simulink model "testSFunctionBuilder"  (R2016a)
settings: Solver=ode1  StartTime=0.0  StopTime=10  FixedStep=0.001  RelTol=1e-3
PostLoadFcn:
  | , if any(exist('dsrtsu_mdlpostloadfcn', 'file') == [2, 3, 6]), try dsrtsu_mdlpostloadfcn('Execute', bdroot); catch fprintf('Error in PostLoadFcn (dsrtsu_mdlpostloadfcn) for model "%s":\n %s\n', bdroot, lasterr); end, end,
settings Model: DSRTSU_INTERNAL_RTI_VER=490  DSRTSU_INTERNAL_RTI_TYPE=rti1401  RTICANMMDATA=struct('GeneralSetupData',struct('modelroot','Z:\Workspace\library\TestSFunctionBuilder','generalsettings',struct('filesettings',struct('destfolder',struct('Name','RTICANMM_FILES','Check',1),'buildfolder',struct('Name','.','Check',1),'AbsDestfolder',struct('Name','Z:\Workspace\library\TestSFunctionBuilder\RTICANMM_FILES'),'AbsBuildfolder',struct('Name','Z:\Workspace\library\TestSFunctionBuilder'))),'options',struct('addpaths',1,'rmpaths',1,'addtrcexclusion',logical(1),'cannavigator',struct('checkmonitoring',0),'show_usrtrc',0,'use_usrtrc',0),'advanced',struct('options',[1 1 1 1 1 1 1 1 1 1 1 1 1 1 1 1 1 1 1 1 1 1 1 1 1 1 1 1 1 1 1 1 1 1 1 1 1 1 1 1 1 1 1 1 1 1 1 1 1 1 1 1 1 1 1 1 1 1 1 1 1 1 1 1 1 1 1 1 1 1 1 1 1 1 1 1 1 1 1 1 1 1 1 1 1 1 1 1 1 1 1 1 1 1 1 1 1 1 1 1]),'MPSetup',{{}},'modelname','testSFunctionBuilder','block','testSFunctionBuilder'))  DSRTSU_INTERNAL_RTIFLEXRAYCONFIG=100  DSRTSU_INTERNAL_RTIFPGA=80  Creator=innovacion  LastModifiedBy=innovacion
settings OptimizationCC: BlockReduction=off  OptimizeBlockIOStorage=off  BufferReuse=off  GlobalBufferReuse=off  ExpressionFolding=off  LocalBlockOutputs=off
settings HardwareCC: ProdBitPerPointer=32  ProdLargestAtomicInteger=Integer  ProdEndianess=BigEndian  ProdWordSize=32  ProdHWDeviceType=Custom Processor->Custom  TargetIntDivRoundTo=Zero  TargetEndianess=BigEndian  TargetHWDeviceType=Custom Processor->Custom
settings RTWCC: SystemTargetFile=rti1401.tlc  MakeCommand=make_rti  TemplateMakefile=rti1401.tmf  Description=dSPACE DS1401 Hardware Platform
settings STFCustomTargetCC: ParMdlRefBuildCompliant=on  MatFileLogging=on  GRTInterface=off  SystemTargetFile=rti1401.tlc
settings GRTTargetCC: CompOptLevelCompliant=off  ConcurrentExecutionCompliant=off  GeneratePreprocessorConditionals=Use local settings  CombineOutputUpdateFcns=off  CPPClassGenCompliant=off  UseToolchainInfoCompliant=off

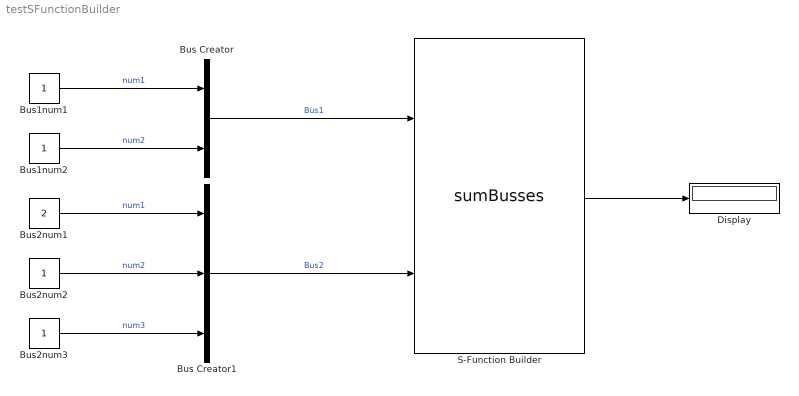
== system testSFunctionBuilder ==
  Bus Creator : BusCreator  Inputs=2  OutDataTypeStr=Bus: Bus1  NonVirtualBus=on
  Bus Creator1 : BusCreator  Inputs=3  OutDataTypeStr=Bus: Bus2  NonVirtualBus=on
  Bus1num1 : Constant  OutDataTypeStr=double
  Bus1num2 : Constant  OutDataTypeStr=double
  Bus2num1 : Constant  Value=2  OutDataTypeStr=double
  Bus2num2 : Constant  OutDataTypeStr=double
  Bus2num3 : Constant  OutDataTypeStr=double
  Display : Display
  S-Function Builder : S-Function  InitFcn=try, set_param(gcb,'FunctionName','sumBusses'), end  FunctionName=sumBusses  SFunctionModules=sumBusses_wrapper  SFunctionDeploymentMode=off  EnableBusSupport=off  mask(S-Function Builder){}
      mask help: Simulink:masks:SFunctionBuilder_MD
      mask init:
      | val = [[.9  0.75 0.75 1 1 .9 .9 1]',[1 1 0.75 0.75 .9 .9 1 .9]'];try , sys = get_param(gcb,'SfunBuilderFcnName');if isempty(sys), sys = get_param(gcb,'FunctionName'); end,catch, sys = get_param(gcb,'FunctionName'); end
      settings: CopyFcn=set_param(gcbh,'LinkStatus','none')  PreSaveFcn=try, set_param(gcb,'FunctionName','sumBusses'), end  OpenFcn=sfunctionwizard(gcbh)
      mask Display: plot(val(:,1),val(:,2)),disp(sys), port_label('input',1,'bus1'), port_label('input',2,'bus2'), port_label('output',1,'result')
  wires:
  Bus1num1/1 -> Bus Creator/1  "num1"
  Bus1num2/1 -> Bus Creator/2  "num2"
  Bus2num1/1 -> Bus Creator1/1  "num1"
  Bus2num2/1 -> Bus Creator1/2  "num2"
  Bus Creator/1 -> S-Function Builder/1  "Bus1"
  Bus Creator1/1 -> S-Function Builder/2  "Bus2"
  S-Function Builder/1 -> Display/1
  Bus2num3/1 -> Bus Creator1/3  "num3"
